simulink model "analysis_yawrate"  (R2019b)
settings: Solver=VariableStepAuto  StartTime=0.0  StopTime=140  RelTol=1e-3
values from neighbouring files (symbols this model uses):
  a0 = a11.*a22 - a12.*a21    [coefficien_lateral_accelration.m]    (also in coefficien_sideslip_angre.m; coefficien_turning_trajectory.m; coefficien_yawrate.m)
  a1 = -a11-a22    [coefficien_lateral_accelration.m]    (also in coefficien_sideslip_angre.m; coefficien_turning_trajectory.m; coefficien_yawrate.m)
  b0 = a21.*b11 - a11.*b21    [coefficien_lateral_accelration.m]    (also in coefficien_sideslip_angre.m = a12.*b21 - a22.*b11; coefficien_turning_trajectory.m; coefficien_yawrate.m)
  b1 = a12.*b21 - a22.*b11 + b21    [coefficien_lateral_accelration.m]    (also in coefficien_sideslip_angre.m = b11; coefficien_turning_trajectory.m; coefficien_yawrate.m = b21)
  V = [8.33333333333 16.6666666667 25 33.3333333333 41.6666666667 50]    [block_params.mat]    (also in coefficien.m = [30:30:180]/3.6; coefficien_lateral_accelration.m = V*(1000/(60*60)); coefficien_sideslip_angre.m = V*(1000/(60*60)); coefficien_turning_trajectory.m = V*(1000/(60*60)))
libraries: cstblocks x1
settings Model: Creator=Natsu Nakagawa  LastModifiedBy=Natsu Nakagawa

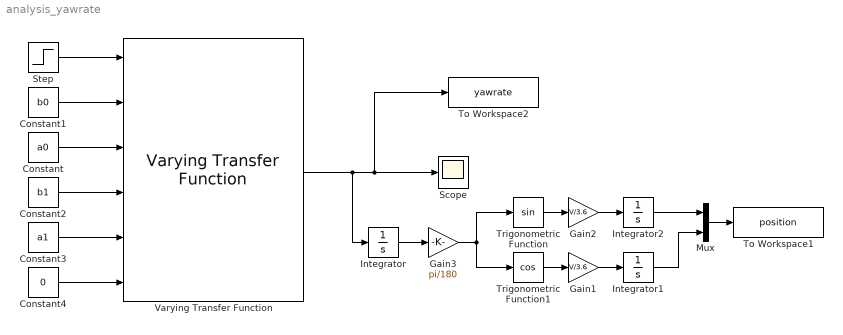
== system analysis_yawrate ==
  Constant : Constant  Value=a0
  Constant1 : Constant  Value=b0
  Constant2 : Constant  Value=b1
  Constant3 : Constant  Value=a1
  Constant4 : Constant  Value=0
  Gain1 : Gain  Gain=V/3.6
  Gain2 : Gain  Gain=V/3.6
  Gain3 : Gain  Gain=pi/180
  Integrator : Integrator
  Integrator1 : Integrator
  Integrator2 : Integrator
  Mux : Mux  Inputs=2
  Scope : Scope
  Step : Step  Time=0  SampleTime=0
  To Workspace1 : ToWorkspace  VariableName=position  SaveFormat=Timeseries  SampleTime=-1
  To Workspace2 : ToWorkspace  VariableName=yawrate  SaveFormat=Timeseries  SampleTime=-1
  Trigonometric Function : Trigonometry
  Trigonometric Function1 : Trigonometry  Operator=cos
  Varying Transfer Function : cstblocks/Linear Parameter Varying/Varying Transfer Function  N=2
      settings: SourceProductName=Control System Toolbox
  wires:
  Step/1 -> Varying Transfer Function/1
  Constant/1 -> Varying Transfer Function/3
  Constant1/1 -> Varying Transfer Function/2
  Constant2/1 -> Varying Transfer Function/4
  Constant3/1 -> Varying Transfer Function/5
  Constant4/1 -> Varying Transfer Function/6
  Integrator/1 -> Gain3/1
  Trigonometric Function1/1 -> Gain1/1
  Integrator2/1 -> Mux/1
  Integrator1/1 -> Mux/2
  Gain3/1 -> Trigonometric Function1/1, Trigonometric Function/1
  Trigonometric Function/1 -> Gain2/1
  Mux/1 -> To Workspace1/1
  Varying Transfer Function/1 -> Integrator/1, Scope/1, To Workspace2/1
  Gain1/1 -> Integrator1/1
  Gain2/1 -> Integrator2/1
